simulink model "UPQC_model"  (R2020b)
settings: Solver=FixedStepAuto  StartTime=0.0  StopTime=Tsim  FixedStep=Tsample  MaxStep=Tsample  RelTol=1e-3
values from neighbouring files (symbols this model uses):
  C_parallel_Series = zeros(1,4)    [Netzmodell_Ini_DL.m]    (also in workspace_Ini.mat = [1e-05 1e-05 1e-05 0])
  C_parallel_Shunt = zeros(1,4)    [Netzmodell_Ini_DL.m]    (also in workspace_Ini.mat = [1e-05 1e-05 1e-05 0])
  CC_Ki = 5    [Netzmodell_Ini_DL.m]    (also in workspace_Ini.mat)
  CC_Ki_geg = 5    [Netzmodell_Ini_DL.m]    (also in workspace_Ini.mat)
  CC_Kp = 10    [Netzmodell_Ini_DL.m]    (also in workspace_Ini.mat)
  CC_Kp_geg = 10    [Netzmodell_Ini_DL.m]    (also in workspace_Ini.mat)
  CC_OS =     [workspace_Ini.mat]
  Czk = Szenario.Czk*u    [Netzmodell_Ini_DL.m]    (also in workspace_Ini.mat = 0.003)
  fak_RVC = Szenario.fak_RVC    [Netzmodell_Ini_DL.m]    (also in workspace_Ini.mat = [1 1 1])
  fak_Uns = [1; 1; 1]    [Netzmodell_Ini_DL.m]    (also in workspace_Ini.mat = [1 1 1])
  Flicker_Schaltzeitpunkte_L1 = Schaltzeitpunkte(1,:)    [Netzmodell_Ini_DL.m]    (also in workspace_Ini.mat = 10.5)
  Flicker_Schaltzeitpunkte_L2 = Schaltzeitpunkte(2,:)    [Netzmodell_Ini_DL.m]    (also in workspace_Ini.mat = 10.5)
  Flicker_Schaltzeitpunkte_L3 = Schaltzeitpunkte(3,:)    [Netzmodell_Ini_DL.m]    (also in workspace_Ini.mat = 10.5)
  fs = [f_nom; f_nom; f_nom]    [Netzmodell_Ini_DL.m]    (also in workspace_Ini.mat = [50 50 50])
  fsw = Szenario.fsw*k    [Netzmodell_Ini_DL.m]    (also in workspace_Ini.mat = 20000)
  I_Basis_Ober_L1 = I_Basis_Ober(1)    [Netzmodell_Ini_DL.m]    (also in workspace_Ini.mat = 0)
  I_Basis_Ober_L2 = I_Basis_Ober(2)    [Netzmodell_Ini_DL.m]    (also in workspace_Ini.mat = 0)
  I_Basis_Ober_L3 = I_Basis_Ober(3)    [Netzmodell_Ini_DL.m]    (also in workspace_Ini.mat = 0)
  I_relativ_Ober_L1 = Szenario.I_relativ_Ober_L1    [Netzmodell_Ini_DL.m]    (also in workspace_Ini.mat = [0 100 0 100 100 0 100 100 0 0 0 0 ... (50 elements, 1x50)])
  I_relativ_Ober_L2 = Szenario.I_relativ_Ober_L2    [Netzmodell_Ini_DL.m]    (also in workspace_Ini.mat = [0 100 0 100 100 0 100 100 0 0 0 0 ... (50 elements, 1x50)])
  I_relativ_Ober_L3 = Szenario.I_relativ_Ober_L3    [Netzmodell_Ini_DL.m]    (also in workspace_Ini.mat = [0 100 0 100 100 0 100 100 0 0 0 0 ... (50 elements, 1x50)])
  L_Ausgang_Series = zeros(1,4)    [Netzmodell_Ini_DL.m]    (also in workspace_Ini.mat = [0.00093 0.00093 0.00093 0.00093])
  L_Ausgang_Shunt = zeros(1,4)    [Netzmodell_Ini_DL.m]    (also in workspace_Ini.mat = [0.00093 0.00093 0.00093 0.00093])
  L_Eingang_Series = zeros(1,4)    [Netzmodell_Ini_DL.m]    (also in workspace_Ini.mat = [0.00085 0.00085 0.00085 0.00085])
  L_Eingang_Shunt = zeros(1,4)    [Netzmodell_Ini_DL.m]    (also in workspace_Ini.mat = [0.00085 0.00085 0.00085 0.00085])
  Ls_in = 52.2*u/10    (= 5.22e-06)    [Netzmodell_Ini_DL.m]    (also in workspace_Ini.mat)
  Ltrans = Szenario.Ltrans*m    [Netzmodell_Ini_DL.m]    (also in workspace_Ini.mat = 0.000256)
  OS_off = 6    [Netzmodell_Ini_DL.m]    (also in workspace_Ini.mat)
  OS_on = 1    [Netzmodell_Ini_DL.m]    (also in workspace_Ini.mat)
  Phi_Ober_L1 = Phi_Ober(1)    [Netzmodell_Ini_DL.m]    (also in workspace_Ini.mat = 0)
  Phi_Ober_L2 = Phi_Ober(2)    [Netzmodell_Ini_DL.m]    (also in workspace_Ini.mat = -120)
  Phi_Ober_L3 = Phi_Ober(3)    [Netzmodell_Ini_DL.m]    (also in workspace_Ini.mat = 120)
  Phis = [0; -120; 120]    [Netzmodell_Ini_DL.m]    (also in workspace_Ini.mat = [0 -120 120])
  Pl_Flicker = Pl_Flicker*k    [Netzmodell_Ini_DL.m]    (also in workspace_Ini.mat = [5000 5000 5000])
  Pl_Grund = Szenario.Pl_Grund *k    [Netzmodell_Ini_DL.m]    (also in workspace_Ini.mat = [5 5 5])
  Pl_RVC = Pl_RVC*k    [Netzmodell_Ini_DL.m]    (also in workspace_Ini.mat = [10000 10000 10000])
  Pl_Uns = Pl_Uns*k    [Netzmodell_Ini_DL.m]    (also in workspace_Ini.mat = [25000 10 10])
  Ql_ind_Flicker = Ql_ind_Flicker*k    [Netzmodell_Ini_DL.m]    (also in workspace_Ini.mat = [0 0 0])
  Ql_ind_Grund = Szenario.Ql_ind_Grund*k    [Netzmodell_Ini_DL.m]    (also in workspace_Ini.mat = [0 0 0])
  Ql_ind_RVC = Szenario.Ql_ind_RVC*k    [Netzmodell_Ini_DL.m]    (also in workspace_Ini.mat = [0 0 0])
  Ql_ind_Uns = Ql_ind_Uns*k    [Netzmodell_Ini_DL.m]    (also in workspace_Ini.mat = [0 0 0])
  Ql_kap_Flicker = Ql_kap_Flicker*k    [Netzmodell_Ini_DL.m]    (also in workspace_Ini.mat = [0 0 0])
  Ql_kap_Grund = Szenario.Ql_kap_Grund*k    [Netzmodell_Ini_DL.m]    (also in workspace_Ini.mat = [0 0 0])
  Ql_kap_RVC = Szenario.Ql_kap_RVC*k    [Netzmodell_Ini_DL.m]    (also in workspace_Ini.mat = [0 0 0])
  Ql_kap_Uns = Ql_kap_Uns*k    [Netzmodell_Ini_DL.m]    (also in workspace_Ini.mat = [0 0 0])
  R_Ausgang_Series = zeros(1,4)    [Netzmodell_Ini_DL.m]    (also in workspace_Ini.mat = [0.1 0.1 0.1 0.1])
  R_Ausgang_Shunt = zeros(1,4)    [Netzmodell_Ini_DL.m]    (also in workspace_Ini.mat = [0.1 0.1 0.1 0.1])
  R_Eingang_Series = zeros(1,4)    [Netzmodell_Ini_DL.m]    (also in workspace_Ini.mat = [0.1 0.1 0.1 0.1])
  R_Eingang_Shunt = zeros(1,4)    [Netzmodell_Ini_DL.m]    (also in workspace_Ini.mat = [0.1 0.1 0.1 0.1])
  R_parallel_Series = zeros(1,4)    [Netzmodell_Ini_DL.m]    (also in workspace_Ini.mat = [13 13 13 0])
  R_parallel_Shunt = zeros(1,4)    [Netzmodell_Ini_DL.m]    (also in workspace_Ini.mat = [13 13 13 0])
  R_ZK_Belastung = 20    [Netzmodell_Ini_DL.m]    (also in workspace_Ini.mat)
  Rs_in = 5.2*m/10    (= 0.00052)    [Netzmodell_Ini_DL.m]    (also in workspace_Ini.mat)
  Rtrans = Szenario.Rtrans    [Netzmodell_Ini_DL.m]    (also in workspace_Ini.mat = 0.206)
  RVC_L1_on_off_Zeitpunkte = Szenario.RVC_L1_on_off_Zeitpunkte    [Netzmodell_Ini_DL.m]    (also in workspace_Ini.mat = [10.5 40 10 11 12 13 14 15])
  RVC_L2_on_off_Zeitpunkte = Szenario.RVC_L2_on_off_Zeitpunkte    [Netzmodell_Ini_DL.m]    (also in workspace_Ini.mat = [10.5 40 10 11 12 13 14 15])
  RVC_L3_on_off_Zeitpunkte = Szenario.RVC_L3_on_off_Zeitpunkte    [Netzmodell_Ini_DL.m]    (also in workspace_Ini.mat = [10.5 40 10 11 12 13 14 15])
  RVC_off = 20.5    [Netzmodell_Ini_DL.m]    (also in workspace_Ini.mat)
  RVC_on = 20    [Netzmodell_Ini_DL.m]    (also in workspace_Ini.mat)
  RVC_val = [0.8,0.8,0.8]    [Netzmodell_Ini_DL.m]    (also in workspace_Ini.mat = [0.8 0.8 0.8])
  strans = Szenario.strans    [Netzmodell_Ini_DL.m]    (also in workspace_Ini.mat = 0.25)
  t_breaker_series = tacts    [Netzmodell_Ini_DL.m]    (also in workspace_Ini.mat = 0.5)
  tact = Szenario.tact    [Netzmodell_Ini_DL.m]    (also in workspace_Ini.mat = 0.5)
  tact_OS_Regler = Szenario.tact_OS_Regler    [Netzmodell_Ini_DL.m]    (also in workspace_Ini.mat = 0.5)
  tact_QU = 10    [Netzmodell_Ini_DL.m]    (also in workspace_Ini.mat)
  tacts = Szenario.tacts    [Netzmodell_Ini_DL.m]    (also in workspace_Ini.mat = 0.5)
  Tsample = Szenario.Tsample    [Netzmodell_Ini_DL.m]    (also in workspace_Ini.mat = 5e-06)
  Uns_L1_on_off_Zeitpunkte = Szenario.Uns_L1_on_off_Zeitpunkte    [Netzmodell_Ini_DL.m]    (also in workspace_Ini.mat = [1 6 10 11 12 13 14 15])
  Uns_L2_on_off_Zeitpunkte = Szenario.Uns_L2_on_off_Zeitpunkte    [Netzmodell_Ini_DL.m]    (also in workspace_Ini.mat = [10 30 10 11 12 13 14 15])
  Uns_L3_on_off_Zeitpunkte = Szenario.Uns_L3_on_off_Zeitpunkte    [Netzmodell_Ini_DL.m]    (also in workspace_Ini.mat = [10 30 10 11 12 13 14 15])
  Us = [Us_Amp; Us_Amp; Us_Amp]    [Netzmodell_Ini_DL.m]    (also in workspace_Ini.mat = [326.598632371 326.598632371 326.598632371])
  Us_Amp = sqrt(2)*400/sqrt(3)    [Netzmodell_Ini_DL.m]    (also in workspace_Ini.mat = 326.598632371)
  VC_Ki_gegen = 30    [Netzmodell_Ini_DL.m]    (also in workspace_Ini.mat)
  VC_Ki_gegen_shunt = 15    [Netzmodell_Ini_DL.m]    (also in workspace_Ini.mat)
  VC_Ki_mit = 5    [Netzmodell_Ini_DL.m]    (also in workspace_Ini.mat)
  VC_Kp_gegen = 5    [workspace_Ini.mat]
  VC_Kp_gegen_shunt = 2    [Netzmodell_Ini_DL.m]    (also in workspace_Ini.mat)
  VC_Kp_mit = 10    [Netzmodell_Ini_DL.m]    (also in workspace_Ini.mat)
  VC_ZK_Ki = 5    [Netzmodell_Ini_DL.m]    (also in workspace_Ini.mat)
  VC_ZK_Kp = 0.5    [Netzmodell_Ini_DL.m]    (also in workspace_Ini.mat)
  Vielfache_Ober_L1 = Szenario.Vielfache_Ober_L1    [Netzmodell_Ini_DL.m]    (also in workspace_Ini.mat = [1 2 3 4 5 6 7 8 9 10 11 12 ... (50 elements, 1x50)])
  Vielfache_Ober_L2 = Szenario.Vielfache_Ober_L2    [Netzmodell_Ini_DL.m]    (also in workspace_Ini.mat = [1 2 3 4 5 6 7 8 9 10 11 12 ... (50 elements, 1x50)])
  Vielfache_Ober_L3 = Szenario.Vielfache_Ober_L3    [Netzmodell_Ini_DL.m]    (also in workspace_Ini.mat = [1 2 3 4 5 6 7 8 9 10 11 12 ... (50 elements, 1x50)])
  ZK_Belastung_off = 100    [Netzmodell_Ini_DL.m]    (also in workspace_Ini.mat)
  ZK_Belastung_on = 100    [Netzmodell_Ini_DL.m]    (also in workspace_Ini.mat)
  Zwischenkreisspannung = 700    [Netzmodell_Ini_DL.m]    (also in workspace_Ini.mat)
undefined symbols (not defined in the file or in its folder): LAusgang, RReiheL3
libraries: powerlib x221, powerlib_meascontrol x80, pid_lib x23, eeTransforms x4, eePwmGeneratorTwoLevel x2, dspstat3 x1
(part 2 of 16)

== system UPQC_model/L Filter Series ==
  Series RLC Branch : powerlib/Elements/Series RLC Branch  LConnTagsString=__new0  RConnTagsString=__new0  BranchType=RL  Resistance=REinL1  Inductance=LEinL1  SetiL0=off  InitialCurrent=0  Capacitance=1e-6  Setx0=off  InitialVoltage=0  Measurements=None
  Series RLC Branch3 : powerlib/Elements/Series RLC Branch  LConnTagsString=__new0  RConnTagsString=__new0  BranchType=RL  Resistance=REinL2  Inductance=LEinL2  SetiL0=off  InitialCurrent=0  Capacitance=1e-6  Setx0=off  InitialVoltage=0  Measurements=None
  Series RLC Branch6 : powerlib/Elements/Series RLC Branch  LConnTagsString=__new0  RConnTagsString=__new0  BranchType=RL  Resistance=REinL3  Inductance=LEinL3  SetiL0=off  InitialCurrent=0  Capacitance=1e-6  Setx0=off  InitialVoltage=0  Measurements=None
  Series RLC Branch9 : powerlib/Elements/Series RLC Branch  Commented=on  LConnTagsString=__new0  RConnTagsString=__new0  BranchType=RL  Resistance=REinN  Inductance=LEinN  SetiL0=off  InitialCurrent=0  Capacitance=1e-6  Setx0=off  InitialVoltage=0  Measurements=None
  L1_Ausgang : PMIOPort  Side=Left
  L1_Eingang : PMIOPort  Port=2  Side=Right
  L2_Ausgang : PMIOPort  Port=3  Side=Left
  L2_Eingang : PMIOPort  Port=4  Side=Right
  L3_Eingang : PMIOPort  Port=5  Side=Right
  L3_Ausgang : PMIOPort  Port=6  Side=Left
  N_Ausgang : PMIOPort  Port=7  Side=Left
  N_Eingang : PMIOPort  Port=8  Side=Right
  connections:
  N_Ausgang/RConn1 -- N_Eingang/RConn1
  L3_Ausgang/RConn1 -- Series RLC Branch6/LConn1
  L1_Ausgang/RConn1 -- Series RLC Branch/LConn1
  Series RLC Branch/RConn1 -- L1_Eingang/RConn1
  Series RLC Branch6/RConn1 -- L3_Eingang/RConn1
  L2_Eingang/RConn1 -- Series RLC Branch3/RConn1
  L2_Ausgang/RConn1 -- Series RLC Branch3/LConn1

== system UPQC_model/L Filter Shunt ==
  Series RLC Branch : powerlib/Elements/Series RLC Branch  LConnTagsString=__new0  RConnTagsString=__new0  BranchType=RL  Resistance=REinL1  Inductance=LEinL1  SetiL0=off  InitialCurrent=0  Capacitance=1e-6  Setx0=off  InitialVoltage=0  Measurements=None
  Series RLC Branch3 : powerlib/Elements/Series RLC Branch  LConnTagsString=__new0  RConnTagsString=__new0  BranchType=RL  Resistance=REinL2  Inductance=LEinL2  SetiL0=off  InitialCurrent=0  Capacitance=1e-6  Setx0=off  InitialVoltage=0  Measurements=None
  Series RLC Branch6 : powerlib/Elements/Series RLC Branch  LConnTagsString=__new0  RConnTagsString=__new0  BranchType=RL  Resistance=REinL3  Inductance=LEinL3  SetiL0=off  InitialCurrent=0  Capacitance=1e-6  Setx0=off  InitialVoltage=0  Measurements=None
  Series RLC Branch9 : powerlib/Elements/Series RLC Branch  Commented=on  LConnTagsString=__new0  RConnTagsString=__new0  BranchType=RL  Resistance=REinN  Inductance=LEinN  SetiL0=off  InitialCurrent=0  Capacitance=1e-6  Setx0=off  InitialVoltage=0  Measurements=None
  L1_Ausgang : PMIOPort  Side=Left
  L1_Eingang : PMIOPort  Port=2  Side=Right
  L2_Ausgang : PMIOPort  Port=3  Side=Left
  L2_Eingang : PMIOPort  Port=4  Side=Right
  L3_Eingang : PMIOPort  Port=5  Side=Right
  L3_Ausgang : PMIOPort  Port=6  Side=Left
  N_Ausgang : PMIOPort  Port=7  Side=Left
  N_Eingang : PMIOPort  Port=8  Side=Right
  connections:
  N_Ausgang/RConn1 -- N_Eingang/RConn1
  L3_Ausgang/RConn1 -- Series RLC Branch6/LConn1
  L1_Ausgang/RConn1 -- Series RLC Branch/LConn1
  Series RLC Branch/RConn1 -- L1_Eingang/RConn1
  Series RLC Branch6/RConn1 -- L3_Eingang/RConn1
  L2_Eingang/RConn1 -- Series RLC Branch3/RConn1
  L2_Ausgang/RConn1 -- Series RLC Branch3/LConn1

== system UPQC_model/LC Filter Series ==
  Current Measurement : powerlib/Measurements/Current Measurement  PhasorSimulation=off  OutputType=Complex  PSBequivalent=0
  Current Measurement1 : powerlib/Measurements/Current Measurement  PhasorSimulation=off  OutputType=Complex  PSBequivalent=0
  Current Measurement2 : powerlib/Measurements/Current Measurement  PhasorSimulation=off  OutputType=Complex  PSBequivalent=0
  Ground : powerlib/Elements/Ground  LConnTagsString=a
  LC_Series_U_I_Scope : Scope  NumInputPorts=2
  LC_Series_para_V : Scope
  Mux : Mux  Inputs=3
  Mux1 : Mux  Inputs=3
  Series RLC Branch1 : powerlib/Elements/Series RLC Branch  LConnTagsString=__new0  RConnTagsString=__new0  BranchType=RC  Resistance=RReiheL1  Inductance=LAusgang  SetiL0=off  InitialCurrent=0  Capacitance=CL1  Setx0=off  InitialVoltage=0  Measurements=None
  Series RLC Branch2 : powerlib/Elements/Series RLC Branch  LConnTagsString=__new0  RConnTagsString=__new0  BranchType=RC  Resistance=RReiheL1  Inductance=LAusgang  SetiL0=off  InitialCurrent=0  Capacitance=CL1  Setx0=off  InitialVoltage=0  Measurements=None
  Series RLC Branch3 : powerlib/Elements/Series RLC Branch  LConnTagsString=__new0  RConnTagsString=__new0  BranchType=RL  Resistance=REinL1  Inductance=LEinL1  SetiL0=off  InitialCurrent=0  Capacitance=1e-6  Setx0=off  InitialVoltage=0  Measurements=None
  Series RLC Branch5 : powerlib/Elements/Series RLC Branch  LConnTagsString=__new0  RConnTagsString=__new0  BranchType=RL  Resistance=REinL1  Inductance=LEinL1  SetiL0=off  InitialCurrent=0  Capacitance=1e-6  Setx0=off  InitialVoltage=0  Measurements=None
  Series RLC Branch6 : powerlib/Elements/Series RLC Branch  LConnTagsString=__new0  RConnTagsString=__new0  BranchType=RC  Resistance=RReiheL1  Inductance=LAusgang  SetiL0=off  InitialCurrent=0  Capacitance=CL1  Setx0=off  InitialVoltage=0  Measurements=None
  Series RLC Branch7 : powerlib/Elements/Series RLC Branch  LConnTagsString=__new0  RConnTagsString=__new0  BranchType=RL  Resistance=REinL1  Inductance=LEinL1  SetiL0=off  InitialCurrent=0  Capacitance=1e-6  Setx0=off  InitialVoltage=0  Measurements=None
  Series RLC Branch9 : powerlib/Elements/Series RLC Branch  Commented=on  LConnTagsString=__new0  RConnTagsString=__new0  BranchType=RL  Resistance=REinN  Inductance=LEinN  SetiL0=off  InitialCurrent=0  Capacitance=1e-6  Setx0=off  InitialVoltage=0  Measurements=None
  Voltage Measurement{,1..3} (4 alike) : powerlib/Measurements/Voltage Measurement  PhasorSimulation=off  OutputType=Complex  PSBequivalent=0
  L1_Ausgang : PMIOPort  Side=Left
  L1_Eingang : PMIOPort  Port=2  Side=Right
  L2_Ausgang : PMIOPort  Port=3  Side=Left
  L2_Eingang : PMIOPort  Port=4  Side=Right
  L3_Eingang : PMIOPort  Port=5  Side=Right
  L3_Ausgang : PMIOPort  Port=6  Side=Left
  N_Ausgang : PMIOPort  Port=7  Side=Left
  N_Eingang : PMIOPort  Port=8  Side=Right
  wires:
  Current Measurement/1 -> Mux/1
  Current Measurement2/1 -> Mux/2
  Current Measurement1/1 -> Mux/3
  Voltage Measurement/1 -> LC_Series_para_V/1
  Voltage Measurement1/1 -> Mux1/1
  Voltage Measurement2/1 -> Mux1/2
  Voltage Measurement3/1 -> Mux1/3
  Mux1/1 -> LC_Series_U_I_Scope/2
  Mux/1 -> LC_Series_U_I_Scope/1
  connections:
  N_Eingang/RConn1 -- N_Ausgang/RConn1
  Series RLC Branch1/LConn1 -- Voltage Measurement2/LConn1 -- L2_Ausgang/RConn1 -- Series RLC Branch5/RConn1
  L1_Eingang/RConn1 -- Current Measurement/LConn1
  Series RLC Branch5/LConn1 -- L2_Eingang/RConn1
  L3_Eingang/RConn1 -- Series RLC Branch3/LConn1
  Current Measurement/RConn1 -- Series RLC Branch7/LConn1
  Current Measurement1/RConn1 -- Voltage Measurement/LConn1 -- Series RLC Branch2/LConn1
  Current Measurement2/RConn1 -- Voltage Measurement1/LConn1 -- L1_Ausgang/RConn1
  Current Measurement2/LConn1 -- Current Measurement1/LConn1 -- Series RLC Branch7/RConn1
  L3_Ausgang/RConn1 -- Voltage Measurement3/LConn1 -- Series RLC Branch3/RConn1 -- Series RLC Branch6/LConn1
  Ground/LConn1 -- Voltage Measurement1/LConn2 -- Voltage Measurement3/LConn2 -- Voltage Measurement2/LConn2
  Series RLC Branch6/RConn1 -- Voltage Measurement/LConn2 -- Series RLC Branch2/RConn1 -- Series RLC Branch1/RConn1

== system UPQC_model/LC Filter Shunt ==
  Current Measurement : powerlib/Measurements/Current Measurement  PhasorSimulation=off  OutputType=Complex  PSBequivalent=0
  Current Measurement1 : powerlib/Measurements/Current Measurement  PhasorSimulation=off  OutputType=Complex  PSBequivalent=0
  Current Measurement2 : powerlib/Measurements/Current Measurement  PhasorSimulation=off  OutputType=Complex  PSBequivalent=0
  LC_Shunt_U_I_Scope : Scope  NumInputPorts=4
  Series RLC Branch : powerlib/Elements/Series RLC Branch  LConnTagsString=__new0  RConnTagsString=__new0  BranchType=RL  Resistance=REinL1  Inductance=LEinL1  SetiL0=off  InitialCurrent=0  Capacitance=1e-6  Setx0=off  InitialVoltage=0  Measurements=None
  Series RLC Branch1 : powerlib/Elements/Series RLC Branch  LConnTagsString=__new0  RConnTagsString=__new0  BranchType=RC  Resistance=RReiheL1  Inductance=LAusgang  SetiL0=off  InitialCurrent=0  Capacitance=CL1  Setx0=off  InitialVoltage=0  Measurements=None
  Series RLC Branch11 : powerlib/Elements/Series RLC Branch  LConnTagsString=__new0  RConnTagsString=__new0  BranchType=RC  Resistance=RReiheL3  Inductance=2.4e-3  SetiL0=off  InitialCurrent=0  Capacitance=CL3  Setx0=off  InitialVoltage=0  Measurements=None
  Series RLC Branch3 : powerlib/Elements/Series RLC Branch  LConnTagsString=__new0  RConnTagsString=__new0  BranchType=RL  Resistance=REinL2  Inductance=LEinL2  SetiL0=off  InitialCurrent=0  Capacitance=1e-6  Setx0=off  InitialVoltage=0  Measurements=None
  Series RLC Branch4 : powerlib/Elements/Series RLC Branch  LConnTagsString=__new0  RConnTagsString=__new0  BranchType=RC  Resistance=RReiheL2  Inductance=2.4e-3  SetiL0=off  InitialCurrent=0  Capacitance=CL2  Setx0=off  InitialVoltage=0  Measurements=None
  Series RLC Branch6 : powerlib/Elements/Series RLC Branch  LConnTagsString=__new0  RConnTagsString=__new0  BranchType=RL  Resistance=REinL3  Inductance=LEinL3  SetiL0=off  InitialCurrent=0  Capacitance=1e-6  Setx0=off  InitialVoltage=0  Measurements=None
  Series RLC Branch9 : powerlib/Elements/Series RLC Branch  Commented=on  LConnTagsString=__new0  RConnTagsString=__new0  BranchType=RL  Resistance=REinN  Inductance=LEinN  SetiL0=off  InitialCurrent=0  Capacitance=1e-6  Setx0=off  InitialVoltage=0  Measurements=None
  Voltage Measurement : powerlib/Measurements/Voltage Measurement  PhasorSimulation=off  OutputType=Complex  PSBequivalent=0
  L1_Ausgang : PMIOPort  Side=Left
  L1_Eingang : PMIOPort  Port=2  Side=Right
  L2_Ausgang : PMIOPort  Port=3  Side=Left
  L2_Eingang : PMIOPort  Port=4  Side=Right
  L3_Eingang : PMIOPort  Port=5  Side=Right
  L3_Ausgang : PMIOPort  Port=6  Side=Left
  N_Ausgang : PMIOPort  Port=7  Side=Left
  N_Eingang : PMIOPort  Port=8  Side=Right
  wires:
  Voltage Measurement/1 -> LC_Shunt_U_I_Scope/1
  Current Measurement/1 -> LC_Shunt_U_I_Scope/2
  Current Measurement1/1 -> LC_Shunt_U_I_Scope/3
  Current Measurement2/1 -> LC_Shunt_U_I_Scope/4
  connections:
  Series RLC Branch11/RConn1 -- Current Measurement/LConn1 -- Voltage Measurement/LConn2
  L3_Ausgang/RConn1 -- Current Measurement2/LConn1
  Series RLC Branch1/LConn1 -- L1_Ausgang/RConn1 -- Series RLC Branch/LConn1
  Series RLC Branch/RConn1 -- L1_Eingang/RConn1
  L2_Ausgang/RConn1 -- Series RLC Branch3/LConn1 -- Series RLC Branch4/LConn1
  Current Measurement1/RConn1 -- L3_Eingang/RConn1
  L2_Eingang/RConn1 -- Series RLC Branch3/RConn1
  Current Measurement/RConn1 -- Series RLC Branch1/RConn1 -- N_Ausgang/RConn1 -- Series RLC Branch4/RConn1 -- N_Eingang/RConn1
  Current Measurement1/LConn1 -- Series RLC Branch6/RConn1
  Voltage Measurement/LConn1 -- Current Measurement2/RConn1 -- Series RLC Branch6/LConn1 -- Series RLC Branch11/LConn1

== system UPQC_model/LCL Filter Series ==
  Current Measurement : powerlib/Measurements/Current Measurement  PhasorSimulation=off  OutputType=Complex  PSBequivalent=0
  Current Measurement1 : powerlib/Measurements/Current Measurement  PhasorSimulation=off  OutputType=Complex  PSBequivalent=0
  Current Measurement2 : powerlib/Measurements/Current Measurement  PhasorSimulation=off  OutputType=Complex  PSBequivalent=0
  Ground : powerlib/Elements/Ground  Commented=on  LConnTagsString=a
  LCL_Series_Scope : Scope  NumInputPorts=2
  Mux : Mux  Inputs=3
  Mux1 : Mux  Inputs=3
  Series RLC Branch : powerlib/Elements/Series RLC Branch  LConnTagsString=__new0  RConnTagsString=__new0  BranchType=RL  Resistance=REinL1  Inductance=LEinL1  SetiL0=off  InitialCurrent=0  Capacitance=1e-6  Setx0=off  InitialVoltage=0  Measurements=None
  Series RLC Branch1 : powerlib/Elements/Series RLC Branch  LConnTagsString=__new0  RConnTagsString=__new0  BranchType=RC  Resistance=RReiheL1  Inductance=LAusgang  SetiL0=off  InitialCurrent=0  Capacitance=CL1  Setx0=off  InitialVoltage=0  Measurements=None
  Series RLC Branch11 : powerlib/Elements/Series RLC Branch  LConnTagsString=__new0  RConnTagsString=__new0  BranchType=RC  Resistance=RReiheL3  Inductance=2.4e-3  SetiL0=off  InitialCurrent=0  Capacitance=CL3  Setx0=off  InitialVoltage=0  Measurements=None
  Series RLC Branch2 : powerlib/Elements/Series RLC Branch  LConnTagsString=__new0  RConnTagsString=__new0  BranchType=RL  Resistance=RAusL1  Inductance=LAusL1  SetiL0=off  InitialCurrent=0  Capacitance=1e-6  Setx0=off  InitialVoltage=0  Measurements=None
  Series RLC Branch3 : powerlib/Elements/Series RLC Branch  LConnTagsString=__new0  RConnTagsString=__new0  BranchType=RL  Resistance=REinL2  Inductance=LEinL2  SetiL0=off  InitialCurrent=0  Capacitance=1e-6  Setx0=off  InitialVoltage=0  Measurements=None
  Series RLC Branch4 : powerlib/Elements/Series RLC Branch  LConnTagsString=__new0  RConnTagsString=__new0  BranchType=RC  Resistance=RReiheL2  Inductance=2.4e-3  SetiL0=off  InitialCurrent=0  Capacitance=CL2  Setx0=off  InitialVoltage=0  Measurements=None
  Series RLC Branch5 : powerlib/Elements/Series RLC Branch  LConnTagsString=__new0  RConnTagsString=__new0  BranchType=RL  Resistance=RAusL2  Inductance=LAusL2  SetiL0=off  InitialCurrent=0  Capacitance=1e-6  Setx0=off  InitialVoltage=0  Measurements=None
  Series RLC Branch6 : powerlib/Elements/Series RLC Branch  LConnTagsString=__new0  RConnTagsString=__new0  BranchType=RL  Resistance=REinL3  Inductance=LEinL3  SetiL0=off  InitialCurrent=0  Capacitance=1e-6  Setx0=off  InitialVoltage=0  Measurements=None
  Series RLC Branch8 : powerlib/Elements/Series RLC Branch  LConnTagsString=__new0  RConnTagsString=__new0  BranchType=RL  Resistance=RAusL3  Inductance=LAusL3  SetiL0=off  InitialCurrent=0  Capacitance=1e-6  Setx0=off  InitialVoltage=0  Measurements=None
  Voltage Measurement : powerlib/Measurements/Voltage Measurement  Commented=on  PhasorSimulation=off  OutputType=Complex  PSBequivalent=0
  Voltage Measurement1 : powerlib/Measurements/Voltage Measurement  Commented=on  PhasorSimulation=off  OutputType=Complex  PSBequivalent=0
  Voltage Measurement2 : powerlib/Measurements/Voltage Measurement  Commented=on  PhasorSimulation=off  OutputType=Complex  PSBequivalent=0
  L1_Ausgang : PMIOPort  Side=Left
  L1_Eingang : PMIOPort  Port=2  Side=Right
  L2_Ausgang : PMIOPort  Port=3  Side=Left
  L2_Eingang : PMIOPort  Port=4  Side=Right
  L3_Eingang : PMIOPort  Port=5  Side=Right
  L3_Ausgang : PMIOPort  Port=6  Side=Left
  N_Ausgang : PMIOPort  Port=7  Side=Left
  N_Eingang : PMIOPort  Port=8  Side=Right
  wires:
  Voltage Measurement1/1 -> Mux1/2
  Current Measurement/1 -> Mux/1
  Voltage Measurement/1 -> Mux1/3
  Mux/1 -> LCL_Series_Scope/1
  Mux1/1 -> LCL_Series_Scope/2
  Voltage Measurement2/1 -> Mux1/1
  Current Measurement2/1 -> Mux/3
  Current Measurement1/1 -> Mux/2
  connections:
  Current Measurement2/LConn1 -- Series RLC Branch1/RConn1
  L3_Ausgang/RConn1 -- Series RLC Branch8/LConn1
  Current Measurement/RConn1 -- Series RLC Branch2/LConn1
  L1_Eingang/RConn1 -- Current Measurement1/RConn1 -- Voltage Measurement2/LConn1
  Series RLC Branch2/RConn1 -- Series RLC Branch1/LConn1 -- Series RLC Branch/LConn1
  Series RLC Branch4/LConn1 -- Series RLC Branch5/RConn1 -- Series RLC Branch3/LConn1
  Series RLC Branch6/RConn1 -- Voltage Measurement/LConn1 -- L3_Eingang/RConn1
  L2_Eingang/RConn1 -- Voltage Measurement1/LConn1 -- Series RLC Branch3/RConn1
  L2_Ausgang/RConn1 -- Series RLC Branch5/LConn1
  Series RLC Branch6/LConn1 -- Series RLC Branch8/RConn1 -- Series RLC Branch11/LConn1
  L1_Ausgang/RConn1 -- Current Measurement/LConn1
  Ground/LConn1 -- Voltage Measurement2/LConn2 -- Voltage Measurement1/LConn2 -- Voltage Measurement/LConn2
  Series RLC Branch/RConn1 -- Current Measurement1/LConn1
  Series RLC Branch4/RConn1 -- Current Measurement2/RConn1 -- Series RLC Branch11/RConn1 -- N_Ausgang/RConn1 -- N_Eingang/RConn1

== system UPQC_model/LCL Filter Shunt ==
  Series RLC Branch : powerlib/Elements/Series RLC Branch  LConnTagsString=__new0  RConnTagsString=__new0  BranchType=RL  Resistance=REinL1  Inductance=LEinL1  SetiL0=off  InitialCurrent=0  Capacitance=1e-6  Setx0=off  InitialVoltage=0  Measurements=None
  Series RLC Branch1 : powerlib/Elements/Series RLC Branch  LConnTagsString=__new0  RConnTagsString=__new0  BranchType=RC  Resistance=RReiheL1  Inductance=LAusgang  SetiL0=off  InitialCurrent=0  Capacitance=CL1  Setx0=off  InitialVoltage=0  Measurements=None
  Series RLC Branch10 : powerlib/Elements/Series RLC Branch  Commented=on  LConnTagsString=__new0  RConnTagsString=__new0  BranchType=RL  Resistance=RAusN  Inductance=LAusN  SetiL0=off  InitialCurrent=0  Capacitance=1e-6  Setx0=off  InitialVoltage=0  Measurements=None
  Series RLC Branch11 : powerlib/Elements/Series RLC Branch  LConnTagsString=__new0  RConnTagsString=__new0  BranchType=RC  Resistance=RReiheL3  Inductance=2.4e-3  SetiL0=off  InitialCurrent=0  Capacitance=CL3  Setx0=off  InitialVoltage=0  Measurements=None
  Series RLC Branch2 : powerlib/Elements/Series RLC Branch  LConnTagsString=__new0  RConnTagsString=__new0  BranchType=RL  Resistance=RAusL1  Inductance=LAusL1  SetiL0=off  InitialCurrent=0  Capacitance=1e-6  Setx0=off  InitialVoltage=0  Measurements=None
  Series RLC Branch3 : powerlib/Elements/Series RLC Branch  LConnTagsString=__new0  RConnTagsString=__new0  BranchType=RL  Resistance=REinL2  Inductance=LEinL2  SetiL0=off  InitialCurrent=0  Capacitance=1e-6  Setx0=off  InitialVoltage=0  Measurements=None
  Series RLC Branch4 : powerlib/Elements/Series RLC Branch  LConnTagsString=__new0  RConnTagsString=__new0  BranchType=RC  Resistance=RReiheL2  Inductance=2.4e-3  SetiL0=off  InitialCurrent=0  Capacitance=CL2  Setx0=off  InitialVoltage=0  Measurements=None
  Series RLC Branch5 : powerlib/Elements/Series RLC Branch  LConnTagsString=__new0  RConnTagsString=__new0  BranchType=RL  Resistance=RAusL2  Inductance=LAusL2  SetiL0=off  InitialCurrent=0  Capacitance=1e-6  Setx0=off  InitialVoltage=0  Measurements=None
  Series RLC Branch6 : powerlib/Elements/Series RLC Branch  LConnTagsString=__new0  RConnTagsString=__new0  BranchType=RL  Resistance=REinL3  Inductance=LEinL3  SetiL0=off  InitialCurrent=0  Capacitance=1e-6  Setx0=off  InitialVoltage=0  Measurements=None
  Series RLC Branch8 : powerlib/Elements/Series RLC Branch  LConnTagsString=__new0  RConnTagsString=__new0  BranchType=RL  Resistance=RAusL3  Inductance=LAusL3  SetiL0=off  InitialCurrent=0  Capacitance=1e-6  Setx0=off  InitialVoltage=0  Measurements=None
  Series RLC Branch9 : powerlib/Elements/Series RLC Branch  Commented=on  LConnTagsString=__new0  RConnTagsString=__new0  BranchType=RL  Resistance=REinN  Inductance=LEinN  SetiL0=off  InitialCurrent=0  Capacitance=1e-6  Setx0=off  InitialVoltage=0  Measurements=None
  L1_Ausgang : PMIOPort  Side=Left
  L1_Eingang : PMIOPort  Port=2  Side=Right
  L2_Ausgang : PMIOPort  Port=3  Side=Left
  L2_Eingang : PMIOPort  Port=4  Side=Right
  L3_Eingang : PMIOPort  Port=5  Side=Right
  L3_Ausgang : PMIOPort  Port=6  Side=Left
  N_Ausgang : PMIOPort  Port=7  Side=Left
  N_Eingang : PMIOPort  Port=8  Side=Right
  connections:
  N_Eingang/RConn1 -- N_Ausgang/RConn1 -- Series RLC Branch11/RConn1 -- Series RLC Branch4/RConn1 -- Series RLC Branch1/RConn1
  L3_Ausgang/RConn1 -- Series RLC Branch8/LConn1
  L1_Ausgang/RConn1 -- Series RLC Branch2/LConn1
  Series RLC Branch/RConn1 -- L1_Eingang/RConn1
  Series RLC Branch2/RConn1 -- Series RLC Branch1/LConn1 -- Series RLC Branch/LConn1
  Series RLC Branch4/LConn1 -- Series RLC Branch3/LConn1 -- Series RLC Branch5/RConn1
  Series RLC Branch6/RConn1 -- L3_Eingang/RConn1
  L2_Eingang/RConn1 -- Series RLC Branch3/RConn1
  L2_Ausgang/RConn1 -- Series RLC Branch5/LConn1
  Series RLC Branch6/LConn1 -- Series RLC Branch11/LConn1 -- Series RLC Branch8/RConn1

== system UPQC_model/Leitungsnachbildung RL ==
  Series RLC Branch{,1..3} (4 alike) : powerlib/Elements/Series RLC Branch  LConnTagsString=__new0  RConnTagsString=__new0  BranchType=RL  Resistance=R_pro_KM*KM  Inductance=L_pro_KM*KM  SetiL0=off  InitialCurrent=0  Capacitance=1e-6  Setx0=off  InitialVoltage=0  Measurements=None
  L1_In : PMIOPort  Side=Left
  L1_Out : PMIOPort  Port=2  Side=Right
  L2_In : PMIOPort  Port=3  Side=Left
  L2_Out : PMIOPort  Port=4  Side=Right
  L3_In : PMIOPort  Port=5  Side=Left
  L3_Out : PMIOPort  Port=6  Side=Right
  N_In : PMIOPort  Port=7  Side=Left
  N_Out : PMIOPort  Port=8  Side=Right
  connections:
  Series RLC Branch/LConn1 -- L1_In/RConn1
  Series RLC Branch/RConn1 -- L1_Out/RConn1
  Series RLC Branch1/RConn1 -- L2_Out/RConn1
  Series RLC Branch1/LConn1 -- L2_In/RConn1
  Series RLC Branch2/LConn1 -- L3_In/RConn1
  Series RLC Branch2/RConn1 -- L3_Out/RConn1
  N_In/RConn1 -- Series RLC Branch3/LConn1
  Series RLC Branch3/RConn1 -- N_Out/RConn1

== system UPQC_model/Leitungsnachbildung RL1 ==
  Series RLC Branch{,1..3} (4 alike) : powerlib/Elements/Series RLC Branch  LConnTagsString=__new0  RConnTagsString=__new0  BranchType=RL  Resistance=R_pro_KM*KM  Inductance=L_pro_KM*KM  SetiL0=off  InitialCurrent=0  Capacitance=1e-6  Setx0=off  InitialVoltage=0  Measurements=None
  L1_In : PMIOPort  Side=Left
  L1_Out : PMIOPort  Port=2  Side=Right
  L2_In : PMIOPort  Port=3  Side=Left
  L2_Out : PMIOPort  Port=4  Side=Right
  L3_In : PMIOPort  Port=5  Side=Left
  L3_Out : PMIOPort  Port=6  Side=Right
  N_In : PMIOPort  Port=7  Side=Left
  N_Out : PMIOPort  Port=8  Side=Right
  connections:
  Series RLC Branch/LConn1 -- L1_In/RConn1
  Series RLC Branch/RConn1 -- L1_Out/RConn1
  Series RLC Branch1/RConn1 -- L2_Out/RConn1
  Series RLC Branch1/LConn1 -- L2_In/RConn1
  Series RLC Branch2/LConn1 -- L3_In/RConn1
  Series RLC Branch2/RConn1 -- L3_Out/RConn1
  N_In/RConn1 -- Series RLC Branch3/LConn1
  Series RLC Branch3/RConn1 -- N_Out/RConn1

== system UPQC_model/Measurement Transformer ==
  Ground4 : powerlib/Elements/Ground  LConnTagsString=a
  Mux : Mux  Inputs=3
  Trafo_NetzseitigSig_Scope : Scope
  U_A__GRD_netz_trafo_Scope : Scope  NumInputPorts=3
  U_B__GRD_netz_trafo_Scope : Scope  NumInputPorts=3
  U_C__GRD_netz_trafo_Scope : Scope  NumInputPorts=3
  Voltage Measurement{,1..9,14} (11 alike) : powerlib/Measurements/Voltage Measurement  PhasorSimulation=off  OutputType=Complex  PSBequivalent=0
  + : PMIOPort  Side=Left
  +1 : PMIOPort  Port=2  Side=Left
  - : PMIOPort  Port=3  Side=Left
  -1 : PMIOPort  Port=4  Side=Left
  +2 : PMIOPort  Port=5  Side=Left
  -2 : PMIOPort  Port=6  Side=Left
  wires:
  Voltage Measurement2/1 -> Mux/3
  Voltage Measurement3/1 -> U_A__GRD_netz_trafo_Scope/1
  Voltage Measurement/1 -> U_A__GRD_netz_trafo_Scope/2, Mux/1
  Voltage Measurement6/1 -> U_B__GRD_netz_trafo_Scope/3
  Voltage Measurement1/1 -> Mux/2
  Voltage Measurement8/1 -> U_C__GRD_netz_trafo_Scope/2
  Voltage Measurement14/1 -> U_A__GRD_netz_trafo_Scope/3
  Mux/1 -> Trafo_NetzseitigSig_Scope/1
  Voltage Measurement4/1 -> U_B__GRD_netz_trafo_Scope/1
  Voltage Measurement5/1 -> U_B__GRD_netz_trafo_Scope/2
  Voltage Measurement7/1 -> U_C__GRD_netz_trafo_Scope/1
  Voltage Measurement9/1 -> U_C__GRD_netz_trafo_Scope/3
  connections:
  Voltage Measurement7/LConn1 -- Voltage Measurement9/LConn2 -- +2/RConn1 -- Voltage Measurement2/LConn1
  Voltage Measurement3/LConn1 -- Voltage Measurement/LConn1 -- +/RConn1
  Voltage Measurement5/LConn1 -- Voltage Measurement6/LConn1 -- -1/RConn1 -- Voltage Measurement1/LConn2
  -2/RConn1 -- Voltage Measurement2/LConn2 -- Voltage Measurement8/LConn1 -- Voltage Measurement9/LConn1
  Voltage Measurement4/LConn1 -- Voltage Measurement1/LConn1 -- Voltage Measurement6/LConn2 -- -/RConn1
  Voltage Measurement8/LConn2 -- Voltage Measurement5/LConn2 -- Voltage Measurement14/LConn2 -- Voltage Measurement3/LConn2 -- Voltage Measurement4/LConn2 -- Voltage Measurement7/LConn2 -- Ground4/LConn1
  Voltage Measurement/LConn2 -- Voltage Measurement14/LConn1 -- +1/RConn1

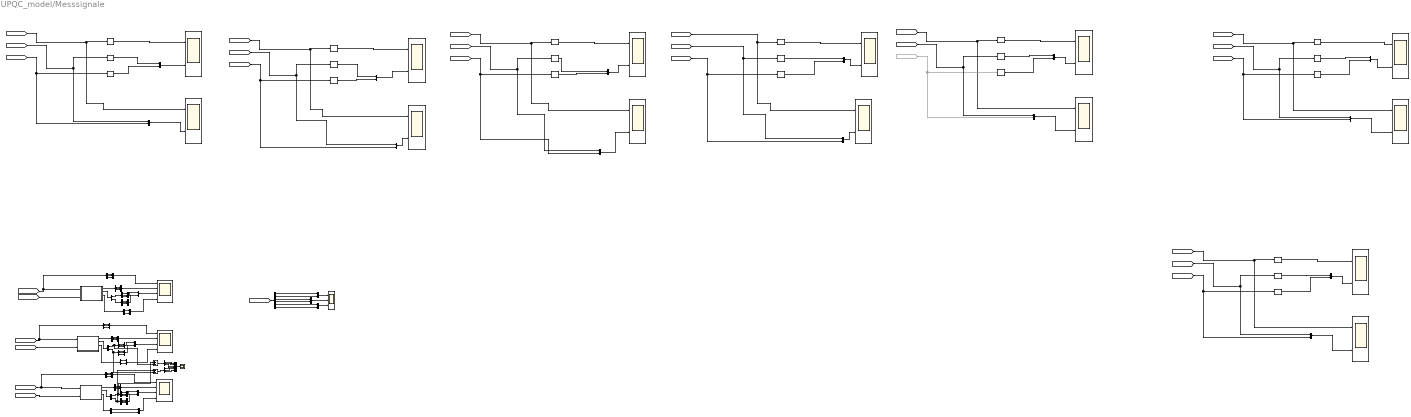
== system UPQC_model/Messsignale ==
  note: (G) Messung Last und Leitung
  note: (G) Messung Zwischenkreis
  note: (F) Unsymmetrie und Leistung
  note: Zeit
  note: (B) Messung UPQC
  note: (A) Messung Ortsnetzstation
  note: (C) Messung hinter UPQC
  note: (D) Messung Shunt UPQC
  note: (E) Messung Series UPQC
  note: RMS
  note: Zeit
  note: RMS
  note: Zeit
  note: RMS Shunt
  note: Zeit
  note: RMS
  note: Zeit
  note: RMS E
  note: Zeit
  note: RMS H
  note: (H) Messung Last
  note: Zeit
  note: RMS G
  A : Subsystem
  A1 : Subsystem
  Bneu : Subsystem
  Bus Creator{,1,3..4,6..7,9..10,12..13,15..16} (12 alike) : BusCreator  Inputs=3
  Bus Creator{2,5,8,11,14,17,19} (7 alike) : BusCreator  Inputs=2
  Bus Creator18 : BusCreator  Inputs=6
  Bus Selector : BusSelector  OutputSignals=U DC Zwischenkreis1,U DC Zwischenkreis2,I DC in1,I DC out1,I DC in2,I DC out2
  Demux{,2..3,5..6,8..9,11..12,14..15,17..19} (14 alike) : Demux  Outputs=3
  Demux{1,4,7,10,13,16} (6 alike) : Demux  Outputs=2
  From33 : From  Commented=on  GotoTag=In_E  TagVisibility=global
  I E : Mux  Inputs=2
  I G : Mux  Inputs=2
  I H : Mux  Inputs=2
  Knoten A : Scope  NumInputPorts=4
  Knoten B : Scope  NumInputPorts=4
  Knoten G : Scope  NumInputPorts=4
  Messung_Zwischenkreis : Scope  NumInputPorts=3
  Mux{,1..11,13} (13 alike) : Mux  Inputs=2
  PQ UPQC : Scope
  Pc-Pb : Sum  Inputs=+-
  Qc-Qb : Sum  Inputs=+-
  RMS A : Scope  NumInputPorts=2
  RMS B : Scope  NumInputPorts=2
  RMS C : Scope  NumInputPorts=2
  RMS D : Scope  NumInputPorts=2
  RMS E : Scope  NumInputPorts=2
  RMS G : Scope  NumInputPorts=2
  RMS H : Scope  NumInputPorts=2
  RMS I_A : powerlib_meascontrol/Measurements/RMS  TrueRMS=on  Freq=50  RMSInit=0  Ts=0
  RMS I_C : powerlib_meascontrol/Measurements/RMS  TrueRMS=on  Freq=50  RMSInit=0  Ts=0
  RMS I_C neu B : powerlib_meascontrol/Measurements/RMS  TrueRMS=on  Freq=50  RMSInit=0  Ts=0
  RMS I_D : powerlib_meascontrol/Measurements/RMS  TrueRMS=on  Freq=50  RMSInit=0  Ts=0
  RMS I_E : powerlib_meascontrol/Measurements/RMS  TrueRMS=on  Freq=50  RMSInit=0  Ts=0
  RMS I_G : powerlib_meascontrol/Measurements/RMS  TrueRMS=on  Freq=50  RMSInit=0  Ts=0
  RMS I_H : powerlib_meascontrol/Measurements/RMS  TrueRMS=on  Freq=50  RMSInit=0  Ts=0
  RMS N A : powerlib_meascontrol/Measurements/RMS  TrueRMS=on  Freq=50  RMSInit=0  Ts=0
  RMS N C : powerlib_meascontrol/Measurements/RMS  TrueRMS=on  Freq=50  RMSInit=0  Ts=0
  RMS N C neu B : powerlib_meascontrol/Measurements/RMS  TrueRMS=on  Freq=50  RMSInit=0  Ts=0
  RMS N D : powerlib_meascontrol/Measurements/RMS  TrueRMS=on  Freq=50  RMSInit=0  Ts=0
  RMS N E : powerlib_meascontrol/Measurements/RMS  TrueRMS=on  Freq=50  RMSInit=0  Ts=0
  RMS N G : powerlib_meascontrol/Measurements/RMS  TrueRMS=on  Freq=50  RMSInit=0  Ts=0
  RMS N H : powerlib_meascontrol/Measurements/RMS  TrueRMS=on  Freq=50  RMSInit=0  Ts=0
  RMS U_A : powerlib_meascontrol/Measurements/RMS  TrueRMS=on  Freq=50  RMSInit=0  Ts=0
  RMS U_C : powerlib_meascontrol/Measurements/RMS  TrueRMS=on  Freq=50  RMSInit=0  Ts=0
  RMS U_C neu B : powerlib_meascontrol/Measurements/RMS  TrueRMS=on  Freq=50  RMSInit=0  Ts=0
  RMS U_D : powerlib_meascontrol/Measurements/RMS  TrueRMS=on  Freq=50  RMSInit=0  Ts=0
  RMS U_E : powerlib_meascontrol/Measurements/RMS  TrueRMS=on  Freq=50  RMSInit=0  Ts=0
  RMS U_G : powerlib_meascontrol/Measurements/RMS  TrueRMS=on  Freq=50  RMSInit=0  Ts=0
  RMS U_H : powerlib_meascontrol/Measurements/RMS  TrueRMS=on  Freq=50  RMSInit=0  Ts=0
  Zeit A : Scope  NumInputPorts=2
  Zeit B : Scope  NumInputPorts=2
  Zeit C : Scope  NumInputPorts=2
  Zeit D : Scope  NumInputPorts=2
  Zeit E : Scope  NumInputPorts=2
  Zeit G : Scope  NumInputPorts=2
  Zeit H : Scope  NumInputPorts=2
  wires:
  [Iabc_A] -> RMS I_A/1, Mux10/1
  [In_A] -> Mux10/2, RMS N A/1
  [Vabc_A] -> Zeit A/1, RMS U_A/1
  RMS I_A/1 -> Mux11/1
  RMS N A/1 -> Mux11/2
  RMS I_C/1 -> Mux8/1
  RMS N C/1 -> Mux8/2
  RMS U_C/1 -> RMS C/1
  [Iabc_C] -> RMS I_C/1, Mux9/1
  [In_C] -> Mux9/2, RMS N C/1
  [Vabc_C] -> Zeit C/1, RMS U_C/1
  [In_B] -> Mux7/2, RMS N C neu B/1
  [Vabc_B] -> Zeit B/1, RMS U_C neu B/1
  RMS U_C neu B/1 -> RMS B/1
  [Iabc_B] -> RMS I_C neu B/1, Mux7/1
  RMS I_D/1 -> Mux4/1
  [Iabc_D] -> Mux6/1, RMS I_D/1
  RMS N D/1 -> Mux4/2
  RMS U_D/1 -> RMS D/1
  [Vabc_D] -> Zeit D/1, RMS U_D/1
  [In_D] -> Mux6/2, RMS N D/1
  [Vabc_E] -> Zeit E/1, RMS U_E/1
  From33/1 -> I E/2, RMS N E/1
  RMS U_E/1 -> RMS E/1
  [Iabc_E] -> RMS I_E/1, I E/1
  RMS N E/1 -> Mux3/2
  RMS I_E/1 -> Mux3/1
  [Vabc_A] -> A/1(Vabc), Demux/1  "Vabc"
  [Iabc_A] -> A/2(I)
  Demux5/1 -> Bus Creator/1  "+"
  Demux5/2 -> Bus Creator/2  "-"
  Demux5/3 -> Bus Creator/3  "0"
  Bus Creator/1 -> Knoten A/2
  Bus Creator1/1 -> Knoten A/1
  Demux/1 -> Bus Creator1/1  "Va"
  Demux/2 -> Bus Creator1/2  "Vb"
  Demux/3 -> Bus Creator1/3  "Vc"
  Demux1/1 -> Bus Creator2/1  "kU2"
  Demux1/2 -> Bus Creator2/2  "kU0"
  Bus Creator2/1 -> Knoten A/4
  Demux3/2 -> Bus Creator4/2  "Q2"
  Bus Creator3/1 -> Bus Creator5/1
  Bus Creator4/1 -> Bus Creator5/2
  Demux3/3 -> Bus Creator4/3  "Q3"
  Demux2/2 -> Bus Creator3/2  "P2"
  Demux3/1 -> Bus Creator4/1  "Q1"
  Demux2/1 -> Bus Creator3/1  "P1"
  Demux2/3 -> Bus Creator3/3  "P3"
  A/2(PQ) -> Demux4/1  "PQ"
  Demux4/1 -> Demux2/1
  Demux4/2 -> Demux3/1
  Bus Creator5/1 -> Knoten A/3
  A/1(+-0 normiert) -> Demux5/1  "+-0"
  A/3(kU2,kU0) -> Demux1/1  "kU2, kU0"
  Bneu/3("kU2, kU0") -> Demux7/1  "kU2, kU0"
  Bus Creator11/1 -> Knoten G/3
  Bus Creator10/1 -> Bus Creator11/2
  Bus Creator7/1 -> Knoten G/1
  Demux6/3 -> Bus Creator7/3  "Vc"
  Demux10/1 -> Pc-Pb/2, Demux8/1
  Demux9/1 -> Bus Creator10/1  "Q1"
  Bus Creator6/1 -> Knoten G/2
  Demux8/2 -> Bus Creator9/2  "P2"
  Demux8/1 -> Bus Creator9/1  "P1"
  Demux9/3 -> Bus Creator10/3  "Q3"
  Demux8/3 -> Bus Creator9/3  "P3"
  Demux9/2 -> Bus Creator10/2  "Q2"
  Bneu/2(PQ) -> Demux10/1  "PQ"
  Demux6/1 -> Bus Creator7/1  "Va"
  [Vabc_G] -> Demux6/1, Bneu/1(Vabc)  "Vabc"
  [Iabc_G] -> Bneu/2(I)
  Bneu/1(+-0 normiert) -> Demux11/1  "+-0"
  Demux10/2 -> Qc-Qb/2, Demux9/1
  Bus Creator9/1 -> Bus Creator11/1
  Demux7/1 -> Bus Creator8/1  "kU2"
  Demux7/2 -> Bus Creator8/2  "kU0"
  Demux6/2 -> Bus Creator7/2  "Vb"
  Demux11/3 -> Bus Creator6/3  "0"
  Demux11/2 -> Bus Creator6/2  "-"
  Bus Creator8/1 -> Knoten G/4
  Demux11/1 -> Bus Creator6/1  "+"
  A1/3("kU2, kU0") -> Demux13/1  "kU2, kU0"
  Bus Creator17/1 -> Knoten B/3
  Bus Creator16/1 -> Bus Creator17/2
  Bus Creator13/1 -> Knoten B/1
  Demux12/3 -> Bus Creator13/3  "Vc"
  Demux16/1 -> Pc-Pb/1, Demux14/1
  Demux15/1 -> Bus Creator16/1  "Q1"
  Bus Creator12/1 -> Knoten B/2
  Demux14/2 -> Bus Creator15/2  "P2"
  Demux14/1 -> Bus Creator15/1  "P1"
  Demux15/3 -> Bus Creator16/3  "Q3"
  Demux14/3 -> Bus Creator15/3  "P3"
  Demux15/2 -> Bus Creator16/2  "Q2"
  A1/2(PQ) -> Demux16/1  "PQ"
  Demux12/1 -> Bus Creator13/1  "Va"
  [Vabc_B] -> Demux12/1, A1/1(Vabc)  "Vabc"
  [Iabc_B] -> A1/2(I)
  A1/1(+-0 normiert) -> Demux17/1  "+-0"
  Demux16/2 -> Qc-Qb/1, Demux15/1
  Bus Creator15/1 -> Bus Creator17/1
  Demux13/2 -> Bus Creator14/2  "kU0"
  Demux12/2 -> Bus Creator13/2  "Vb"
  Demux17/3 -> Bus Creator12/3  "0"
  Demux17/2 -> Bus Creator12/2  "-"
  Bus Creator14/1 -> Knoten B/4
  Demux17/1 -> Bus Creator12/1  "+"
  Qc-Qb/1 -> Demux19/1
  Demux18/3 -> Bus Creator18/3  "P3"
  Demux18/2 -> Bus Creator18/2  "P2"
  Pc-Pb/1 -> Demux18/1
  Demux18/1 -> Bus Creator18/1  "P1"
  Demux19/1 -> Bus Creator18/4  "Q1"
  Demux19/2 -> Bus Creator18/5  "Q2"
  Demux19/3 -> Bus Creator18/6  "Q3"
  Bus Creator18/1 -> PQ UPQC/1
  Demux13/1 -> Bus Creator14/1  "kU2"
  [Messung_Zwischenkreis] -> Bus Selector/1
  Bus Selector/1 -> Mux/1  "<U DC Zwischenkreis1>"
  Bus Selector/2 -> Mux/2  "<U DC Zwischenkreis2>"
  Mux/1 -> Messung_Zwischenkreis/1
  Bus Selector/6 -> Mux2/2  "<I DC out2>"
  Mux2/1 -> Messung_Zwischenkreis/3
  Mux1/1 -> Messung_Zwischenkreis/2
  Bus Selector/3 -> Mux1/1  "<I DC in1>"
  Bus Selector/4 -> Mux1/2  "<I DC out1>"
  Bus Selector/5 -> Mux2/1  "<I DC in2>"
  Mux3/1 -> RMS E/2
  I E/1 -> Zeit E/2
  Mux4/1 -> RMS D/2
  Mux6/1 -> Zeit D/2
  Mux7/1 -> Zeit B/2
  Mux9/1 -> Zeit C/2
  Mux8/1 -> RMS C/2
  Mux11/1 -> RMS A/2
  RMS U_A/1 -> RMS A/1
  Mux10/1 -> Zeit A/2
  RMS I_C neu B/1 -> Bus Creator19/1
  RMS N C neu B/1 -> Bus Creator19/2
  Bus Creator19/1 -> RMS B/2
  I H/1 -> Zeit H/2
  [Vabc_H] -> Zeit H/1, RMS U_H/1
  RMS N H/1 -> Mux5/2
  [Iabc_H] -> RMS I_H/1, I H/1
  RMS U_H/1 -> RMS H/1
  [In_H] -> I H/2, RMS N H/1
  Mux5/1 -> RMS H/2
  RMS I_H/1 -> Mux5/1
  RMS I_G/1 -> Mux13/1
  Mux13/1 -> RMS G/2
  [In_G] -> I G/2, RMS N G/1
  [Iabc_G] -> RMS I_G/1, I G/1
  RMS N G/1 -> Mux13/2
  RMS U_G/1 -> RMS G/1
  [Vabc_G] -> Zeit G/1, RMS U_G/1
  I G/1 -> Zeit G/2

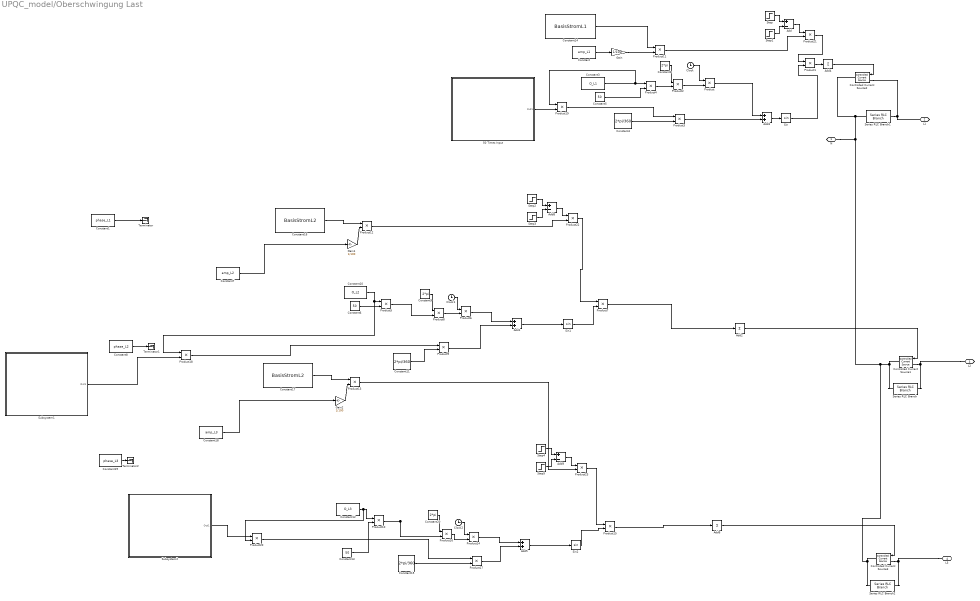
== system UPQC_model/Oberschwingung Last ==
  50 Times Input : Subsystem
  Add : Sum  Inputs=+-
  Add1 : Sum
  Add2 : Sum  Inputs=+
  Add3 : Sum
  Add4 : Sum  Inputs=+
  Add5 : Sum
  Add6 : Sum  Inputs=+
  Add8 : Sum  Inputs=+-
  Add9 : Sum  Inputs=+-
  Clock : Clock
  Clock1 : Clock
  Clock2 : Clock
  Constant : Constant  Value=amp_L1
  Constant1 : Constant  Value=phase_L1
  Constant10 : Constant  Value=O_L2
  Constant11 : Constant  Value=2*pi/360
  Constant12 : Constant  Value=O_L3
  Constant13 : Constant  Value=50
  Constant14 : Constant  Value=BasisStromL1
  Constant15 : Constant  Value=2*pi/360
  Constant16 : Constant  Value=BasisStromL2
  Constant17 : Constant  Value=BasisStromL2
  Constant18 : Constant  Value=amp_L3
  Constant19 : Constant  Value=phase_L3
  Constant2 : Constant  Value=2*pi
  Constant20 : Constant  Value=2*pi
  Constant3 : Constant  Value=O_L1
  Constant4 : Constant  Value=2*pi/360
  Constant5 : Constant  Value=50
  Constant6 : Constant  Value=50
  Constant7 : Constant  Value=amp_L2
  Constant8 : Constant  Value=phase_L2
  Constant9 : Constant  Value=2*pi
  Controlled Current Source1 : powerlib/Electrical Sources/Controlled Current Source  Initialize=on  Source_Type=AC  Amplitude=init_amp_L2  Phase=init_phase_L2  Frequency=init_freq_L2  Measurements=None
  Controlled Current Source2 : powerlib/Electrical Sources/Controlled Current Source  Initialize=on  Source_Type=AC  Amplitude=init_amp_L1  Phase=init_phase_L1  Frequency=init_freq_L1  Measurements=None
  Controlled Current Source3 : powerlib/Electrical Sources/Controlled Current Source  Initialize=on  Source_Type=AC  Amplitude=init_amp_L3  Phase=init_phase_L3  Frequency=init_freq_L3  Measurements=None
  Gain : Gain  Gain=1/100
  Gain1 : Gain  Gain=1/100
  Gain2 : Gain  Gain=1/100
  Product{,1..23} (24 alike) : Product
  Series RLC Branch : powerlib/Elements/Series RLC Branch  LConnTagsString=__new0  RConnTagsString=__new0  BranchType=R  Resistance=100000000  Inductance=1e-3  SetiL0=off  InitialCurrent=0  Capacitance=1e-6  Setx0=off  InitialVoltage=0  Measurements=None
  Series RLC Branch1 : powerlib/Elements/Series RLC Branch  LConnTagsString=__new0  RConnTagsString=__new0  BranchType=R  Resistance=100000000  Inductance=1e-3  SetiL0=off  InitialCurrent=0  Capacitance=1e-6  Setx0=off  InitialVoltage=0  Measurements=None
  Series RLC Branch2 : powerlib/Elements/Series RLC Branch  LConnTagsString=__new0  RConnTagsString=__new0  BranchType=R  Resistance=100000000  Inductance=1e-3  SetiL0=off  InitialCurrent=0  Capacitance=1e-6  Setx0=off  InitialVoltage=0  Measurements=None
  Sin : Trigonometry
  Sin1 : Trigonometry
  Sin2 : Trigonometry
  Step : Step  Time=OS_on  SampleTime=0
  Step1 : Step  Time=OS_off  SampleTime=0
  Step2 : Step  Time=OS_on  SampleTime=0
  Step3 : Step  Time=OS_off  SampleTime=0
  Step4 : Step  Time=OS_on  SampleTime=0
  Step5 : Step  Time=OS_off  SampleTime=0
  Subsystem1 : Subsystem
  Subsystem2 : Subsystem
  Terminator : Terminator
  Terminator1 : Terminator
  Terminator2 : Terminator
  N : PMIOPort  Side=Left
  L1 : PMIOPort  Port=2  Side=Right
  L2 : PMIOPort  Port=3  Side=Right
  L3 : PMIOPort  Port=4  Side=Right
  wires:
  Product23/1 -> Product15/1
  Add9/1 -> Product23/1
  Step5/1 -> Add9/2
  Step4/1 -> Add9/1
  Product22/1 -> Product7/1
  Add8/1 -> Product22/1
  Step3/1 -> Add8/2
  Step2/1 -> Add8/1
  Product21/1 -> Product1/1
  Add/1 -> Product21/1
  Step1/1 -> Add/2
  Step/1 -> Add/1
  Product13/1 -> Product23/2
  Constant17/1 -> Product13/1
  Constant18/1 -> Gain2/1
  Gain2/1 -> Product13/2
  Constant8/1 -> Terminator1/1
  Product12/1 -> Product22/2
  Gain1/1 -> Product12/2
  Constant16/1 -> Product12/1
  Gain/1 -> Product11/2
  Product11/1 -> Product21/2
  Constant14/1 -> Product11/1
  Constant13/1 -> Product10/2
  Product10/1 -> Product16/2
  Constant12/1 -> Product20/2, Product10/1
  Product5/1 -> Product8/2
  Constant10/1 -> Product18/1, Product5/1
  Constant6/1 -> Product5/2
  Product4/1 -> Product2/2
  Constant5/1 -> Product4/2
  Constant3/1 -> Product19/1, Product4/1
  Add2/1 -> Controlled Current Source1/1
  Add6/1 -> Controlled Current Source3/1
  Add4/1 -> Controlled Current Source2/1
  Product15/1 -> Add6/1
  Constant20/1 -> Product16/1
  Add5/1 -> Sin2/1
  Clock2/1 -> Product14/1
  Product14/1 -> Add5/1
  Product17/1 -> Add5/2
  Product16/1 -> Product14/2
  Constant15/1 -> Product17/2
  Constant11/1 -> Product9/2
  Product8/1 -> Product6/2
  Product9/1 -> Add1/2
  Product7/1 -> Add2/1
  Clock1/1 -> Product6/1
  Product6/1 -> Add1/1
  Constant7/1 -> Gain1/1
  Add1/1 -> Sin1/1
  Constant9/1 -> Product8/1
  Product3/1 -> Add3/2
  Product/1 -> Add3/1
  Constant/1 -> Gain/1
  Constant2/1 -> Product2/1
  Add3/1 -> Sin/1
  Clock/1 -> Product/1
  Product1/1 -> Add4/1
  Constant4/1 -> Product3/2
  Product2/1 -> Product/2
  Constant1/1 -> Terminator/1
  Constant19/1 -> Terminator2/1
  Sin/1 -> Product1/2
  Sin1/1 -> Product7/2
  Sin2/1 -> Product15/2
  Product19/1 -> Product3/1
  50 Times Input/1(Out1) -> Product19/2
  Subsystem1/1(Out1) -> Product18/2
  Product18/1 -> Product9/1
  Subsystem2/1(Out1) -> Product20/1
  Product20/1 -> Product17/1
  connections:
  L3/RConn1 -- Controlled Current Source3/LConn1 -- Series RLC Branch2/RConn1
  L2/RConn1 -- Controlled Current Source1/LConn1 -- Series RLC Branch/RConn1
  Controlled Current Source2/LConn1 -- L1/RConn1 -- Series RLC Branch1/RConn1
  N/RConn1 -- Controlled Current Source2/RConn1 -- Series RLC Branch1/LConn1 -- Controlled Current Source1/RConn1 -- Series RLC Branch/LConn1 -- Controlled Current Source3/RConn1 -- Series RLC Branch2/LConn1
